simulink model "crearhuerto"  (R2020b)
settings: Solver=VariableStepAuto  StartTime=0.0  StopTime=10.0  RelTol=1e-3
settings Model: Creator=Jose  LastModifiedBy=Jose

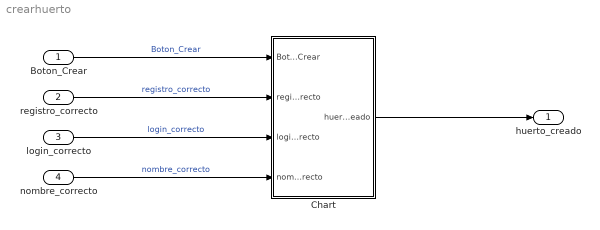
== system crearhuerto ==
  Boton_Crear : Inport  OutDataTypeStr=boolean  PortDimensions=1
  registro_correcto : Inport  Port=2  OutDataTypeStr=boolean  PortDimensions=1
  login_correcto : Inport  Port=3  OutDataTypeStr=boolean  PortDimensions=1
  nombre_correcto : Inport  Port=4  OutDataTypeStr=boolean  PortDimensions=1
  Chart : Stateflow chart  TreatAsAtomicUnit=on
  huerto_creado : Outport  SignalName=huerto_creado  OutDataTypeStr=boolean  PortDimensions=1
      settings: MustResolveToSignalObject=on
  wires:
  Boton_Crear/1 -> Chart/1(Boton_Crear)  "Boton_Crear"
  registro_correcto/1 -> Chart/2(registro_correcto)  "registro_correcto"
  login_correcto/1 -> Chart/3(login_correcto)  "login_correcto"
  nombre_correcto/1 -> Chart/4(nombre_correcto)  "nombre_correcto"
  Chart/1(huerto_creado) -> huerto_creado/1

== stateflow chart crearhuerto/Chart ==
  state OFF
    en:
    huerto_creado=false
  state Comprobar_usuario
    en:
    huerto_creado=false
  note: -1
  state Introducir_nombre
    en:
    huerto_creado=false
  state Huerto_creado
    en:
    huerto_creado=true
  (default) -> OFF
  Comprobar_usuario -> OFF [order 2] : [~registro_correcto]
  Huerto_creado -> OFF [order 1] : [~Boton_Crear]
  OFF -> OFF [order 2] : [~Boton_Crear]
  OFF -> Comprobar_usuario [order 1] : [Boton_Crear==1]
  Huerto_creado -> Comprobar_usuario [order 2] : [Boton_Crear]
  Comprobar_usuario -> Introducir_nombre [order 1] : [registro_correcto]
  Introducir_nombre -> Introducir_nombre [order 2] : [~nombre_correcto]
  Introducir_nombre -> Huerto_creado [order 1] : [nombre_correcto]
  data: Boton_Crear input; registro_correcto input; login_correcto input; nombre_correcto input; huerto_creado output
